simulink model "mavsim_chap10"  (R2020b)
settings: Solver=ode4  StartTime=0.0  StopTime=tsim  FixedStep=P.Ts  RelTol=1e-3  EnableMultiTasking=on
InitFcn:
  | param_chap10
values from neighbouring files (symbols this model uses):
  path_vector = [flag; r; q; chi_inf; k_path; c; rho; lambda; k_orbit]    [pathstruct2pathvec.m]    (also in runSim.m = pathstruct2pathvec(path_struct))
undefined symbols (not defined in the file or in its folder): accelerometer, aileron_c_sat, airspeed, baroAltimeter, calc_chi, closedLoopEnable, elevator_c_sat, forces_moments, get_h, get_p, get_phi, get_q, get_theta, get_Va, gps, gyro, magnetometer, P, phi_c_sat, stateMachine, takeoff_autopilot, theta_c_sat, throttle_c_sat, u_trim, x_trim
libraries: pid_lib x5, simulink x3
settings Model: Creator=beard  LastModifiedBy=alanf
settings DataIOCC: LimitDataPoints=on  SaveFormat=Array  ReturnWorkspaceOutputs=off
settings OptimizationCC: ExpressionDepthLimit=2147483647  InitFltsAndDblsToZero=on  LifeSpan=inf
settings DebuggingCC: UnderspecifiedInitializationDetection=Classic  MergeDetectMultiDrivingBlocksExec=none  SolverPrmCheckMsg=warning  FcnCallInpInsideContextMsg=warning  StateNameClashWarn=warning  SFUnexpectedBacktrackingDiag=warning  SFNoUnconditionalDefaultTransitionDiag=warning  SFExecutionAtInitializationDiag=none  ArithmeticOperatorsInVariantConditions=warning
settings HardwareCC: ProdBitPerPointer=32  ProdBitPerSizeT=32  ProdBitPerPtrDiffT=32  ProdLargestAtomicFloat=None  ProdIntDivRoundTo=Undefined  ProdEndianess=Unspecified  ProdWordSize=32  ProdHWDeviceType=32-bit Generic
settings ModelReferenceCC: PropagateSignalLabelsOutOfModel=off
settings SFSimCC: SimUseLocalCustomCode=off  CustomCodeUndefinedFunction=UseInterfaceOnly
settings RTWCC: RTWUseLocalCustomCode=off
settings CodeAppCC: StateflowObjectComments=on
settings GRTTargetCC: TargetLangStandard=C89/C90 (ANSI)  CombineOutputUpdateFcns=off  GRTInterface=on
settings ConfigComp: CovMetricSettings=dw  CovSaveCumulativeToWorkspaceVar=on  CovSaveSingleToWorkspaceVar=on  CovExternalEMLEnable=off  CovSFcnEnable=off

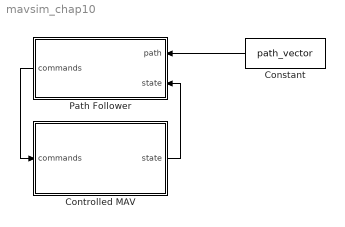
== system mavsim_chap10 ==
  Constant : Constant  Value=path_vector
  Controlled MAV : Subsystem
      mask Display: image(imread('batcam.png'))
  Path Follower : Subsystem
  wires:
  Controlled MAV/1(state) -> Path Follower/2(state)
  Path Follower/1(commands) -> Controlled MAV/1(commands)
  Constant/1 -> Path Follower/1(path)

== system mavsim_chap10/Controlled MAV ==
  commands : Inport
  Autopilot : Subsystem
      mask Display: image(imread('kestrel.jpg'))
  MAV : Subsystem
      mask Display: image(imread('batcam.png'))
  Wind : Subsystem
  state : Outport  VectorParamsAs1DForOutWhenUnconnected=off
  wires:
  Wind/1(Wind) -> MAV/2(wind)
  MAV/1(x) -> state/1, Autopilot/2(x)  "state"
  Autopilot/1(delta) -> MAV/1(delta)
  commands/1 -> Autopilot/1(commands)

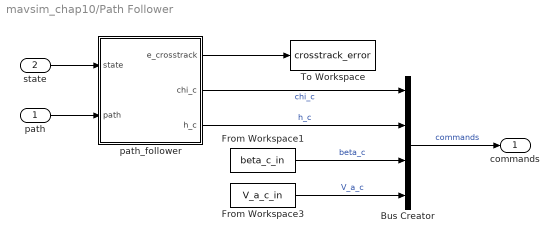
== system mavsim_chap10/Path Follower ==
  path : Inport
  state : Inport  Port=2
  Bus Creator : BusCreator  Inputs=4
  From Workspace1 : FromWorkspace  VariableName=beta_c_in
  From Workspace3 : FromWorkspace  VariableName=V_a_c_in
  To Workspace : ToWorkspace  VariableName=crosstrack_error  SaveFormat=Timeseries  SampleTime=-1
  path_follower : MATLAB Function  TreatAsAtomicUnit=on
  commands : Outport  VectorParamsAs1DForOutWhenUnconnected=off
  wires:
  From Workspace3/1 -> Bus Creator/4  "V_a_c"
  Bus Creator/1 -> commands/1  "commands"
  From Workspace1/1 -> Bus Creator/3  "beta_c"
  path_follower/2(chi_c) -> Bus Creator/1  "chi_c"
  path_follower/3(h_c) -> Bus Creator/2  "h_c"
  state/1 -> path_follower/1(state)
  path/1 -> path_follower/2(path)
  path_follower/1(e_crosstrack) -> To Workspace/1

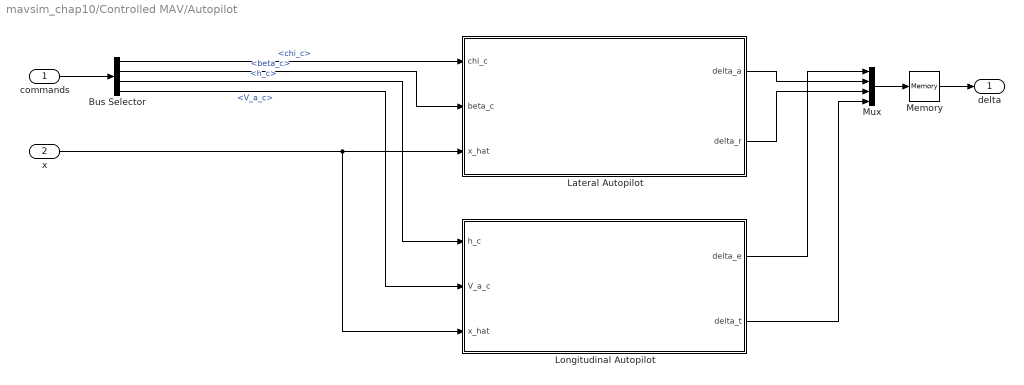
== system mavsim_chap10/Controlled MAV/Autopilot ==
  commands : Inport
  x : Inport  Port=2
  Bus Selector : BusSelector  OutputSignals=chi_c,beta_c,h_c,V_a_c
  Lateral Autopilot : Subsystem
  Longitudinal Autopilot : Subsystem
  Memory : Memory  InitialCondition=P.u_trim  InheritSampleTime=on
  Mux : Mux
  delta : Outport  VectorParamsAs1DForOutWhenUnconnected=off
  wires:
  x/1 -> Longitudinal Autopilot/3(x_hat), Lateral Autopilot/3(x_hat)
  Bus Selector/1 -> Lateral Autopilot/1(chi_c)  "<chi_c>"
  Bus Selector/2 -> Lateral Autopilot/2(beta_c)  "<beta_c>"
  Bus Selector/3 -> Longitudinal Autopilot/1(h_c)  "<h_c>"
  Bus Selector/4 -> Longitudinal Autopilot/2(V_a_c)  "<V_a_c>"
  Mux/1 -> Memory/1
  Memory/1 -> delta/1
  Longitudinal Autopilot/1(delta_e) -> Mux/1
  Lateral Autopilot/1(delta_a) -> Mux/2
  Lateral Autopilot/2(delta_r) -> Mux/3
  Longitudinal Autopilot/2(delta_t) -> Mux/4
  commands/1 -> Bus Selector/1

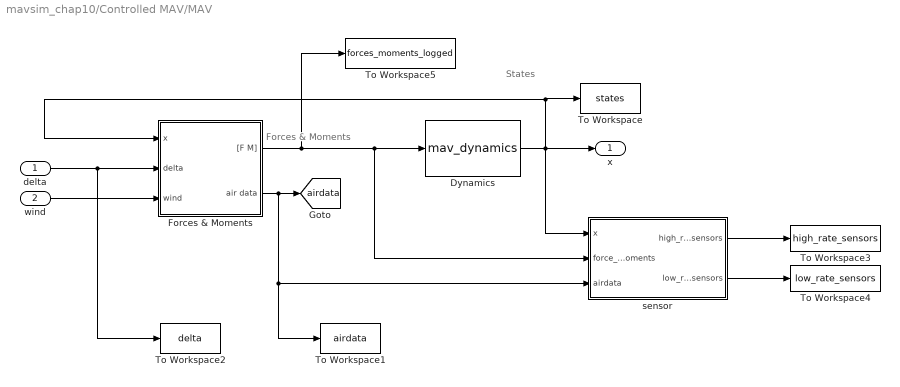
== system mavsim_chap10/Controlled MAV/MAV ==
  note: Forces & Moments
  note: States
  delta : Inport
  wind : Inport  Port=2
  Dynamics : S-Function  FunctionName=mav_dynamics  Parameters=P  SFunctionDeploymentMode=off  EnableBusSupport=off
  Forces & Moments : Subsystem
  To Workspace : ToWorkspace  VariableName=states  SaveFormat=Timeseries  SampleTime=-1
  To Workspace1 : ToWorkspace  VariableName=airdata  SaveFormat=Timeseries  SampleTime=-1
  To Workspace2 : ToWorkspace  VariableName=delta  SaveFormat=Timeseries  SampleTime=-1
  To Workspace3 : ToWorkspace  VariableName=high_rate_sensors  SaveFormat=Timeseries  SampleTime=-1
  To Workspace4 : ToWorkspace  VariableName=low_rate_sensors  SaveFormat=Timeseries  SampleTime=-1
  To Workspace5 : ToWorkspace  VariableName=forces_moments_logged  SaveFormat=Timeseries  SampleTime=-1
  sensor : Subsystem
  x : Outport  VectorParamsAs1DForOutWhenUnconnected=off
  tag scope: airdata=global
  wires:
  Dynamics/1 -> sensor/1(x), Forces & Moments/1(x), To Workspace/1, x/1
  Forces & Moments/1("[F M]") -> To Workspace5/1, sensor/2(force_moments), Dynamics/1
  Forces & Moments/2(air data) -> To Workspace1/1, sensor/3(airdata), [airdata]
  delta/1 -> To Workspace2/1, Forces & Moments/2(delta)
  wind/1 -> Forces & Moments/3(wind)
  sensor/1(high_rate_sensors) -> To Workspace3/1
  sensor/2(low_rate_sensors) -> To Workspace4/1

== system mavsim_chap10/Controlled MAV/Wind ==
  Constant2 : Constant  Value=[P.wind_n; P.wind_e; P.wind_d]
  Mux1 : Mux  Inputs=2
  Wind Gusts : Subsystem
  Wind : Outport  VectorParamsAs1DForOutWhenUnconnected=off
  wires:
  Constant2/1 -> Mux1/1
  Mux1/1 -> Wind/1
  Wind Gusts/1(gusts) -> Mux1/2

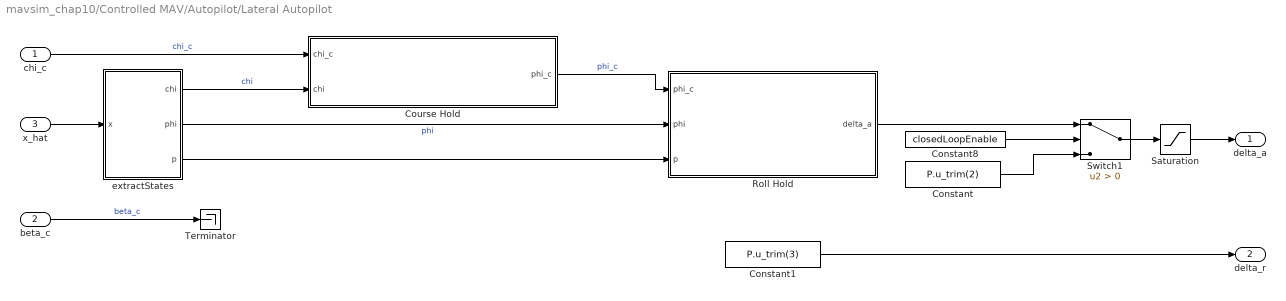
== system mavsim_chap10/Controlled MAV/Autopilot/Lateral Autopilot ==
  chi_c : Inport
  beta_c : Inport  Port=2
  x_hat : Inport  Port=3
  Constant : Constant  Value=P.u_trim(2)
  Constant1 : Constant  Value=P.u_trim(3)
  Constant8 : Constant  Value=closedLoopEnable
  Course Hold : Subsystem
  Roll Hold : Subsystem
  Saturation : Saturate  UpperLimit=aileron_c_sat  LowerLimit=-aileron_c_sat
  Switch1 : Switch  Criteria=u2 > Threshold
  Terminator : Terminator
  extractStates : Subsystem
  delta_a : Outport  VectorParamsAs1DForOutWhenUnconnected=off
  delta_r : Outport  Port=2  VectorParamsAs1DForOutWhenUnconnected=off
  wires:
  chi_c/1 -> Course Hold/1(chi_c)  "chi_c"
  Course Hold/1(phi_c) -> Roll Hold/1(phi_c)  "phi_c"
  x_hat/1 -> extractStates/1(x)
  extractStates/1(chi) -> Course Hold/2(chi)  "chi"
  extractStates/2(phi) -> Roll Hold/2(phi)  "phi"
  extractStates/3(p) -> Roll Hold/3(p)
  Constant1/1 -> delta_r/1
  Switch1/1 -> Saturation/1
  Constant/1 -> Switch1/3
  Roll Hold/1(delta_a) -> Switch1/1
  Constant8/1 -> Switch1/2
  beta_c/1 -> Terminator/1  "beta_c"
  Saturation/1 -> delta_a/1

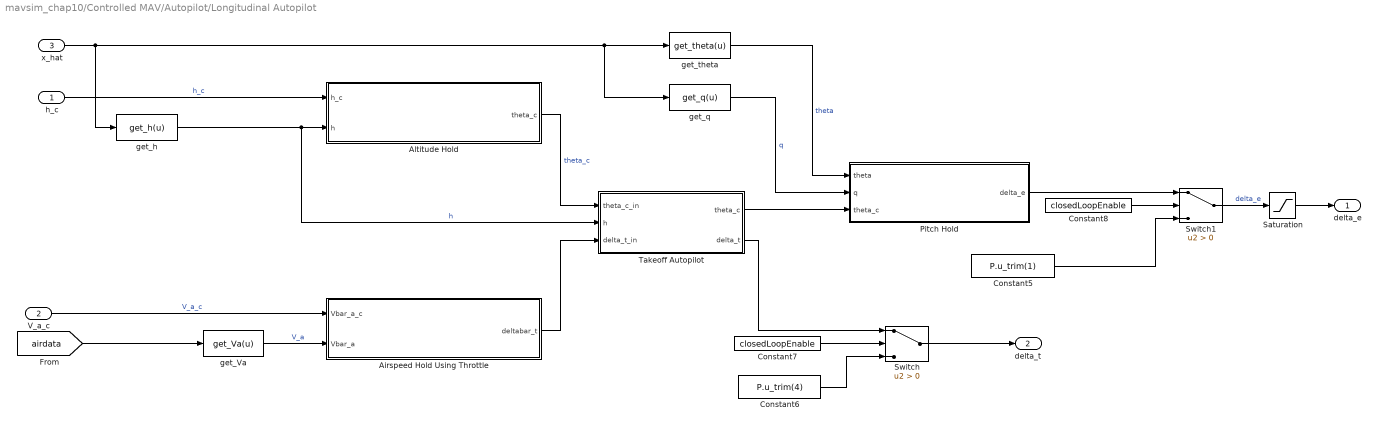
== system mavsim_chap10/Controlled MAV/Autopilot/Longitudinal Autopilot ==
  h_c : Inport
  V_a_c : Inport  Port=2
  x_hat : Inport  Port=3
  Airspeed Hold Using Throttle : Subsystem
  Altitude Hold : Subsystem
  Constant5 : Constant  Value=P.u_trim(1)
  Constant6 : Constant  Value=P.u_trim(4)
  Constant7 : Constant  Value=closedLoopEnable
  Constant8 : Constant  Value=closedLoopEnable
  Pitch Hold : Subsystem
  Saturation : Saturate  UpperLimit=elevator_c_sat  LowerLimit=-elevator_c_sat
  Switch : Switch  Criteria=u2 > Threshold
  Switch1 : Switch  Criteria=u2 > Threshold
  Takeoff Autopilot : Subsystem
  get_Va : MATLABFcn  MATLABFcn=get_Va(u)
  get_h : MATLABFcn  MATLABFcn=get_h(u)
  get_q : MATLABFcn  MATLABFcn=get_q(u)
  get_theta : MATLABFcn  MATLABFcn=get_theta(u)
  delta_e : Outport  VectorParamsAs1DForOutWhenUnconnected=off
  delta_t : Outport  Port=2  VectorParamsAs1DForOutWhenUnconnected=off
  wires:
  h_c/1 -> Altitude Hold/1(h_c)  "h_c"
  x_hat/1 -> get_q/1, get_theta/1, get_h/1
  get_h/1 -> Takeoff Autopilot/2(h), Altitude Hold/2(h)  "h"
  [airdata] -> get_Va/1
  get_Va/1 -> Airspeed Hold Using Throttle/2(Vbar_a)  "V_a"
  get_theta/1 -> Pitch Hold/1(theta)  "theta"
  get_q/1 -> Pitch Hold/2(q)  "q"
  Constant6/1 -> Switch/3
  Switch/1 -> delta_t/1
  Switch1/1 -> Saturation/1  "delta_e"
  Constant5/1 -> Switch1/3
  Constant7/1 -> Switch/2
  Constant8/1 -> Switch1/2
  V_a_c/1 -> Airspeed Hold Using Throttle/1(Vbar_a_c)  "V_a_c"
  Pitch Hold/1(delta_e) -> Switch1/1
  Saturation/1 -> delta_e/1
  Altitude Hold/1(theta_c) -> Takeoff Autopilot/1(theta_c_in)  "theta_c"
  Airspeed Hold Using Throttle/1(deltabar_t) -> Takeoff Autopilot/3(delta_t_in)
  Takeoff Autopilot/1(theta_c) -> Pitch Hold/3(theta_c)
  Takeoff Autopilot/2(delta_t) -> Switch/1

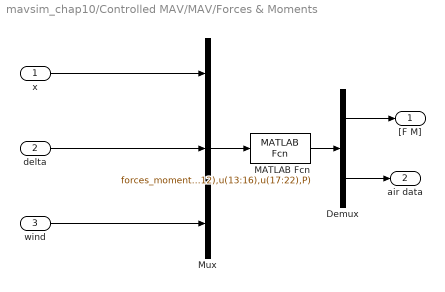
== system mavsim_chap10/Controlled MAV/MAV/Forces & Moments ==
  x : Inport
  delta : Inport  Port=2
  wind : Inport  Port=3
  Demux : Demux  Outputs=[6;6]
  MATLAB Fcn : MATLABFcn  MATLABFcn=forces_moments(u(1:12),u(13:16),u(17:22),P)  OutputDimensions=12
  Mux : Mux  Inputs=3
  "[F M]" : Outport  VectorParamsAs1DForOutWhenUnconnected=off
  air data : Outport  Port=2  VectorParamsAs1DForOutWhenUnconnected=off
  wires:
  Demux/2 -> air data/1
  Mux/1 -> MATLAB Fcn/1
  Demux/1 -> "[F M]"/1
  MATLAB Fcn/1 -> Demux/1
  wind/1 -> Mux/3
  delta/1 -> Mux/2
  x/1 -> Mux/1

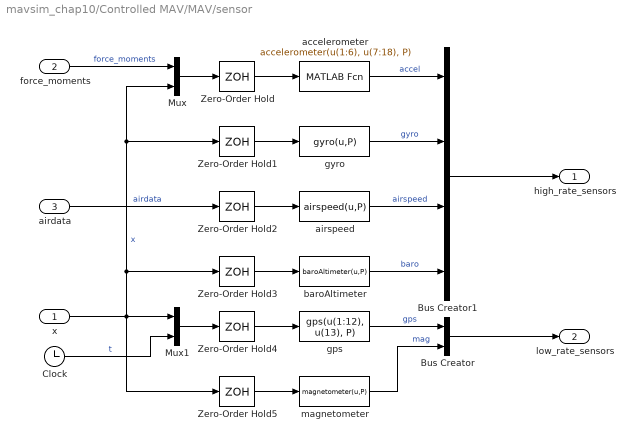
== system mavsim_chap10/Controlled MAV/MAV/sensor ==
  x : Inport
  force_moments : Inport  Port=2
  airdata : Inport  Port=3
  Bus Creator : BusCreator  Inputs=2
  Bus Creator1 : BusCreator  Inputs=4
  Clock : Clock
  Mux : Mux  Inputs=2
  Mux1 : Mux  Inputs=2
  Zero-Order Hold{,1..3} (4 alike) : ZeroOrderHold  SampleTime=P.Ts_highrate
  Zero-Order Hold4 : ZeroOrderHold  SampleTime=P.Ts_lowrate
  Zero-Order Hold5 : ZeroOrderHold  SampleTime=P.Ts_lowrate
  accelerometer : MATLABFcn  MATLABFcn=accelerometer(u(1:6), u(7:18), P)
  airspeed : MATLABFcn  MATLABFcn=airspeed(u,P)
  baroAltimeter : MATLABFcn  MATLABFcn=baroAltimeter(u,P)
  gps : MATLABFcn  MATLABFcn=gps(u(1:12), u(13), P)
  gyro : MATLABFcn  MATLABFcn=gyro(u,P)
  magnetometer : MATLABFcn  MATLABFcn=magnetometer(u,P)
  high_rate_sensors : Outport  VectorParamsAs1DForOutWhenUnconnected=off
  low_rate_sensors : Outport  Port=2  VectorParamsAs1DForOutWhenUnconnected=off
  wires:
  gps/1 -> Bus Creator/1  "gps"
  magnetometer/1 -> Bus Creator/2  "mag"
  Bus Creator/1 -> low_rate_sensors/1
  x/1 -> Mux1/1, Mux/2, Zero-Order Hold1/1, Zero-Order Hold3/1, Zero-Order Hold5/1  "x"
  airdata/1 -> Zero-Order Hold2/1  "airdata"
  accelerometer/1 -> Bus Creator1/1  "accel"
  gyro/1 -> Bus Creator1/2  "gyro"
  airspeed/1 -> Bus Creator1/3  "airspeed"
  baroAltimeter/1 -> Bus Creator1/4  "baro"
  Bus Creator1/1 -> high_rate_sensors/1
  Clock/1 -> Mux1/2  "t"
  Zero-Order Hold/1 -> accelerometer/1
  Zero-Order Hold1/1 -> gyro/1
  Zero-Order Hold2/1 -> airspeed/1
  Zero-Order Hold3/1 -> baroAltimeter/1
  Zero-Order Hold4/1 -> gps/1
  Zero-Order Hold5/1 -> magnetometer/1
  force_moments/1 -> Mux/1  "force_moments"
  Mux/1 -> Zero-Order Hold/1
  Mux1/1 -> Zero-Order Hold4/1

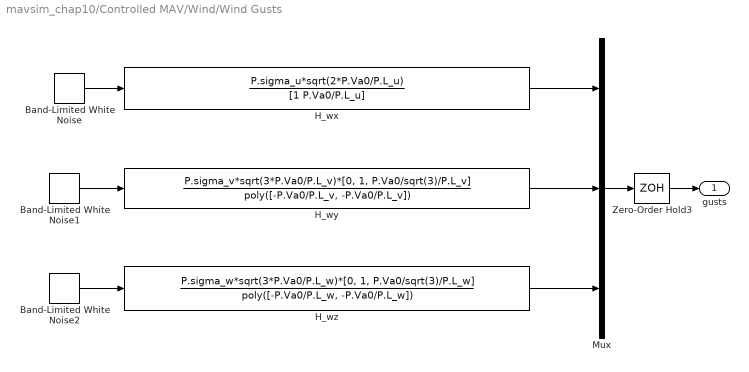
== system mavsim_chap10/Controlled MAV/Wind/Wind Gusts ==
  Band-Limited White Noise : simulink/Sources/Band-Limited White Noise  Cov=[1]  Ts=P.Ts  seed=[23341]
  Band-Limited White Noise1 : simulink/Sources/Band-Limited White Noise  Cov=[1]  Ts=P.Ts  seed=[23341]
  Band-Limited White Noise2 : simulink/Sources/Band-Limited White Noise  Cov=[1]  Ts=P.Ts  seed=[23341]
  H_wx : TransferFcn  Numerator=P.sigma_u*sqrt(2*P.Va0/P.L_u)  Denominator=[1 P.Va0/P.L_u]
  H_wy : TransferFcn  Numerator=P.sigma_v*sqrt(3*P.Va0/P.L_v)*[0, 1, P.Va0/sqrt(3)/P.L_v]  Denominator=poly([-P.Va0/P.L_v, -P.Va0/P.L_v])
  H_wz : TransferFcn  Numerator=P.sigma_w*sqrt(3*P.Va0/P.L_w)*[0, 1, P.Va0/sqrt(3)/P.L_w]  Denominator=poly([-P.Va0/P.L_w, -P.Va0/P.L_w])
  Mux : Mux  Inputs=3
  Zero-Order Hold3 : ZeroOrderHold  SampleTime=P.Ts
  gusts : Outport  VectorParamsAs1DForOutWhenUnconnected=off
  wires:
  H_wx/1 -> Mux/1
  Band-Limited White Noise/1 -> H_wx/1
  H_wy/1 -> Mux/2
  Band-Limited White Noise1/1 -> H_wy/1
  H_wz/1 -> Mux/3
  Band-Limited White Noise2/1 -> H_wz/1
  Mux/1 -> Zero-Order Hold3/1
  Zero-Order Hold3/1 -> gusts/1

== system mavsim_chap10/Controlled MAV/Autopilot/Lateral Autopilot/Course Hold ==
  chi_c : Inport
  chi : Inport  Port=2
  PI Controller : pid_lib/PID Controller  Controller=PI  Form=Parallel  TimeDomain=Continuous-time  UseExternalTs=off  SampleTime=-1  IntegratorMethod=Forward Euler  FilterMethod=Forward Euler  ControllerParametersSource=internal  P=P.k_pchi  I=P.k_ichi  D=0  UseFilter=on  N=100  TunerSelectOption=Transfer Function Based (PID Tuner App)  InitialConditionSource=internal  InitialConditionForIntegrator=x_trim(7)  InitialConditionForFilter=0  DifferentiatorICPrevScaledInput=0  ExternalReset=none  TrackingMode=off  Kt=1  LimitOutput=on  SatLimitsSource=internal  UpperSaturationLimit=phi_c_sat  LowerSaturationLimit=-phi_c_sat  LinearizeAsGain=off  AntiWindupMode=clamping  Kb=1  POutMin=[]  POutMax=[]  IOutMin=[]  IOutMax=[]  DOutMin=[]  DOutMax=[]  NOutMin=[]  NOutMax=[]  SumOutMin=[]  SumOutMax=[]  SaturationOutMin=[]  SaturationOutMax=[]  PParamMin=[]  PParamMax=[]  IParamMin=[]  IParamMax=[]  DParamMin=[]  DParamMax=[]  NParamMin=[]  NParamMax=[]  KbParamMin=[]  KbParamMax=[]  KtParamMin=[]  KtParamMax=[]  KbOutMin=[]  KbOutMax=[]  KtOutMin=[]  KtOutMax=[]  IntegratorOutMin=[]  IntegratorOutMax=[]  FilterOutMin=[]  FilterOutMax=[]  SumI1OutMin=[]  SumI1OutMax=[]  SumI2OutMin=[]  SumI2OutMax=[]  SumI3OutMin=[]  SumI3OutMax=[]  SumI4OutMin=[]  SumI4OutMax=[]  SumDOutMin=[]  SumDOutMax=[]  DifferentiatorOutMin=[]  DifferentiatorOutMax=[]  FilterDiffOutCoefMin=[]  FilterDiffOutCoefMax=[]  ReciprocalOutMin=[]  ReciprocalOutMax=[]  SumDenOutMin=[]  SumDenOutMax=[]  SumNumOutMin=[]  SumNumOutMax=[]  DivideOutMin=[]  DivideOutMax=[]  UdiffTsProdOutMin=[]  UdiffTsProdOutMax=[]  NTsProdOutMin=[]  NTsProdOutMax=[]  UintegralTsProdOutMin=[]  UintegralTsProdOutMax=[]  UngainTsProdOutMin=[]  UngainTsProdOutMax=[]  IntegratorContinuousStateAttributes=''  IntegratorStateMustResolveToSignalObject=off  IntegratorRTWStateStorageClass=Auto  FilterContinuousStateAttributes=''  FilterStateMustResolveToSignalObject=off  FilterRTWStateStorageClass=Auto  ParallelPVariant=InternalParameters  IdealPVariant=Disabled  IVariant=InternalParameters  DVariant=Disabled  IntegratorVariant=Continuous  SatVariant=Enabled  AWVariant=ContClampingParallel  PCopyVariant=Disabled  TRVariant=Disabled  FdbkBlocksVariant=Forward  IdealPFdbkVariant=Disabled  SatFdbkVariant=Disabled  DerivativeFilterVariant=Disabled  NVariant=Disabled  NCopyVariant=Disabled_SignalSpec  FilterICVariant=Disabled  IntegratorICVariant=InternalICs  ExternalResetVariant=Disabled  TRSumVariant=Passthrough  SumFdbkVariant=Disabled  SumVariant=Sum_PI  TsampFilterVariant=InternalTs  TsampNgainVariant=Passthrough  TsampIntegralVariant=Passthrough  ExternalSaturationOutDataTypeStr=Inherit: Same as second input
  Sum1 : Sum  Inputs=|+-
  To Workspace : ToWorkspace  VariableName=chi_c  SaveFormat=Timeseries  SampleTime=-1
  To Workspace1 : ToWorkspace  VariableName=chi  SaveFormat=Timeseries  SampleTime=-1
  phi_c : Outport  VectorParamsAs1DForOutWhenUnconnected=off
  wires:
  chi/1 -> To Workspace1/1, Sum1/2  "chi"
  chi_c/1 -> To Workspace/1, Sum1/1  "chi_c"
  Sum1/1 -> PI Controller/1  "e_chi"
  PI Controller/1 -> phi_c/1

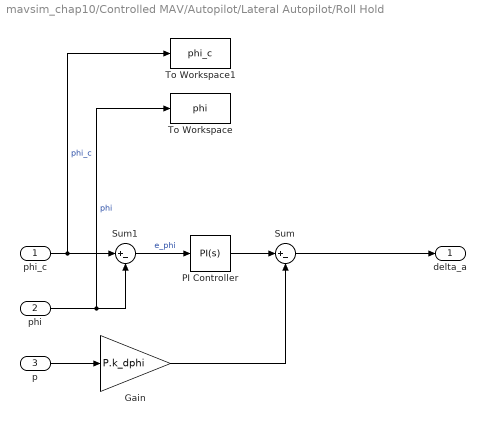
== system mavsim_chap10/Controlled MAV/Autopilot/Lateral Autopilot/Roll Hold ==
  phi_c : Inport
  phi : Inport  Port=2
  p : Inport  Port=3
  Gain : Gain  Gain=P.k_dphi
  PI Controller : pid_lib/PID Controller  Controller=PI  Form=Parallel  TimeDomain=Continuous-time  UseExternalTs=off  SampleTime=-1  IntegratorMethod=Forward Euler  FilterMethod=Forward Euler  ControllerParametersSource=internal  P=P.k_pphi  I=P.k_iphi  D=0  UseFilter=on  N=100  TunerSelectOption=Transfer Function Based (PID Tuner App)  InitialConditionSource=internal  InitialConditionForIntegrator=u_trim(2)  InitialConditionForFilter=0  DifferentiatorICPrevScaledInput=0  ExternalReset=none  TrackingMode=off  Kt=1  LimitOutput=off  SatLimitsSource=internal  UpperSaturationLimit=inf  LowerSaturationLimit=-inf  LinearizeAsGain=on  AntiWindupMode=clamping  Kb=1  POutMin=[]  POutMax=[]  IOutMin=[]  IOutMax=[]  DOutMin=[]  DOutMax=[]  NOutMin=[]  NOutMax=[]  SumOutMin=[]  SumOutMax=[]  SaturationOutMin=[]  SaturationOutMax=[]  PParamMin=[]  PParamMax=[]  IParamMin=[]  IParamMax=[]  DParamMin=[]  DParamMax=[]  NParamMin=[]  NParamMax=[]  KbParamMin=[]  KbParamMax=[]  KtParamMin=[]  KtParamMax=[]  KbOutMin=[]  KbOutMax=[]  KtOutMin=[]  KtOutMax=[]  IntegratorOutMin=[]  IntegratorOutMax=[]  FilterOutMin=[]  FilterOutMax=[]  SumI1OutMin=[]  SumI1OutMax=[]  SumI2OutMin=[]  SumI2OutMax=[]  SumI3OutMin=[]  SumI3OutMax=[]  SumI4OutMin=[]  SumI4OutMax=[]  SumDOutMin=[]  SumDOutMax=[]  DifferentiatorOutMin=[]  DifferentiatorOutMax=[]  FilterDiffOutCoefMin=[]  FilterDiffOutCoefMax=[]  ReciprocalOutMin=[]  ReciprocalOutMax=[]  SumDenOutMin=[]  SumDenOutMax=[]  SumNumOutMin=[]  SumNumOutMax=[]  DivideOutMin=[]  DivideOutMax=[]  UdiffTsProdOutMin=[]  UdiffTsProdOutMax=[]  NTsProdOutMin=[]  NTsProdOutMax=[]  UintegralTsProdOutMin=[]  UintegralTsProdOutMax=[]  UngainTsProdOutMin=[]  UngainTsProdOutMax=[]  IntegratorContinuousStateAttributes=''  IntegratorStateMustResolveToSignalObject=off  IntegratorRTWStateStorageClass=Auto  FilterContinuousStateAttributes=''  FilterStateMustResolveToSignalObject=off  FilterRTWStateStorageClass=Auto  ParallelPVariant=InternalParameters  IdealPVariant=Disabled  IVariant=InternalParameters  DVariant=Disabled  IntegratorVariant=Continuous  SatVariant=Disabled  AWVariant=Passthrough  PCopyVariant=Disabled  TRVariant=Disabled  FdbkBlocksVariant=Forward  IdealPFdbkVariant=Disabled  SatFdbkVariant=Disabled  DerivativeFilterVariant=Disabled  NVariant=Disabled  NCopyVariant=Disabled_SignalSpec  FilterICVariant=Disabled  IntegratorICVariant=InternalICs  ExternalResetVariant=Disabled  TRSumVariant=Passthrough  SumFdbkVariant=Disabled  SumVariant=Sum_PI  TsampFilterVariant=InternalTs  TsampNgainVariant=Passthrough  TsampIntegralVariant=Passthrough  ExternalSaturationOutDataTypeStr=Inherit: Same as second input
  Sum : Sum  Inputs=|+-
  Sum1 : Sum  Inputs=|+-
  To Workspace : ToWorkspace  VariableName=phi  SaveFormat=Timeseries  SampleTime=-1
  To Workspace1 : ToWorkspace  VariableName=phi_c  SaveFormat=Timeseries  SampleTime=-1
  delta_a : Outport  VectorParamsAs1DForOutWhenUnconnected=off
  wires:
  Sum1/1 -> PI Controller/1  "e_phi"
  phi_c/1 -> To Workspace1/1, Sum1/1  "phi_c"
  PI Controller/1 -> Sum/1
  phi/1 -> To Workspace/1, Sum1/2  "phi"
  p/1 -> Gain/1
  Gain/1 -> Sum/2
  Sum/1 -> delta_a/1

== system mavsim_chap10/Controlled MAV/Autopilot/Lateral Autopilot/extractStates ==
  x : Inport
  calc_chi : MATLABFcn  MATLABFcn=calc_chi(u)
  get_p : MATLABFcn  MATLABFcn=get_p(u)
  get_phi : MATLABFcn  MATLABFcn=get_phi(u)
  chi : Outport  VectorParamsAs1DForOutWhenUnconnected=off
  phi : Outport  Port=2  VectorParamsAs1DForOutWhenUnconnected=off
  p : Outport  Port=3  VectorParamsAs1DForOutWhenUnconnected=off
  wires:
  x/1 -> get_p/1, get_phi/1, calc_chi/1
  calc_chi/1 -> chi/1
  get_phi/1 -> phi/1
  get_p/1 -> p/1

== system mavsim_chap10/Controlled MAV/Autopilot/Longitudinal Autopilot/Airspeed Hold Using Throttle ==
  Vbar_a_c : Inport
  Vbar_a : Inport  Port=2
  PI Controller : pid_lib/PID Controller  Controller=PI  Form=Parallel  TimeDomain=Continuous-time  UseExternalTs=off  SampleTime=-1  IntegratorMethod=Forward Euler  FilterMethod=Forward Euler  ControllerParametersSource=internal  P=P.k_pv  I=P.k_iv  D=0  UseFilter=on  N=100  TunerSelectOption=Transfer Function Based (PID Tuner App)  InitialConditionSource=internal  InitialConditionForIntegrator=P.u_trim(4)  InitialConditionForFilter=0  DifferentiatorICPrevScaledInput=0  ExternalReset=none  TrackingMode=off  Kt=1  LimitOutput=on  SatLimitsSource=internal  UpperSaturationLimit=throttle_c_sat  LowerSaturationLimit=0  LinearizeAsGain=on  AntiWindupMode=clamping  Kb=1  POutMin=[]  POutMax=[]  IOutMin=[]  IOutMax=[]  DOutMin=[]  DOutMax=[]  NOutMin=[]  NOutMax=[]  SumOutMin=[]  SumOutMax=[]  SaturationOutMin=[]  SaturationOutMax=[]  PParamMin=[]  PParamMax=[]  IParamMin=[]  IParamMax=[]  DParamMin=[]  DParamMax=[]  NParamMin=[]  NParamMax=[]  KbParamMin=[]  KbParamMax=[]  KtParamMin=[]  KtParamMax=[]  KbOutMin=[]  KbOutMax=[]  KtOutMin=[]  KtOutMax=[]  IntegratorOutMin=[]  IntegratorOutMax=[]  FilterOutMin=[]  FilterOutMax=[]  SumI1OutMin=[]  SumI1OutMax=[]  SumI2OutMin=[]  SumI2OutMax=[]  SumI3OutMin=[]  SumI3OutMax=[]  SumI4OutMin=[]  SumI4OutMax=[]  SumDOutMin=[]  SumDOutMax=[]  DifferentiatorOutMin=[]  DifferentiatorOutMax=[]  FilterDiffOutCoefMin=[]  FilterDiffOutCoefMax=[]  ReciprocalOutMin=[]  ReciprocalOutMax=[]  SumDenOutMin=[]  SumDenOutMax=[]  SumNumOutMin=[]  SumNumOutMax=[]  DivideOutMin=[]  DivideOutMax=[]  UdiffTsProdOutMin=[]  UdiffTsProdOutMax=[]  NTsProdOutMin=[]  NTsProdOutMax=[]  UintegralTsProdOutMin=[]  UintegralTsProdOutMax=[]  UngainTsProdOutMin=[]  UngainTsProdOutMax=[]  IntegratorContinuousStateAttributes=''  IntegratorStateMustResolveToSignalObject=off  IntegratorRTWStateStorageClass=Auto  FilterContinuousStateAttributes=''  FilterStateMustResolveToSignalObject=off  FilterRTWStateStorageClass=Auto  ParallelPVariant=InternalParameters  IdealPVariant=Disabled  IVariant=InternalParameters  DVariant=Disabled  IntegratorVariant=Continuous  SatVariant=Enabled  AWVariant=ContClampingParallel  PCopyVariant=Disabled  TRVariant=Disabled  FdbkBlocksVariant=Forward  IdealPFdbkVariant=Disabled  SatFdbkVariant=Disabled  DerivativeFilterVariant=Disabled  NVariant=Disabled  NCopyVariant=Disabled_SignalSpec  FilterICVariant=Disabled  IntegratorICVariant=InternalICs  ExternalResetVariant=Disabled  TRSumVariant=Passthrough  SumFdbkVariant=Disabled  SumVariant=Sum_PI  TsampFilterVariant=InternalTs  TsampNgainVariant=Passthrough  TsampIntegralVariant=Passthrough  ExternalSaturationOutDataTypeStr=Inherit: Same as second input
  Sum1 : Sum  Inputs=|+-
  To Workspace : ToWorkspace  VariableName=Vbar_a_c  SaveFormat=Timeseries  SampleTime=-1
  To Workspace1 : ToWorkspace  VariableName=Vbar_a  SaveFormat=Timeseries  SampleTime=-1
  deltabar_t : Outport  VectorParamsAs1DForOutWhenUnconnected=off
  wires:
  Sum1/1 -> PI Controller/1
  Vbar_a_c/1 -> To Workspace/1, Sum1/1
  Vbar_a/1 -> To Workspace1/1, Sum1/2
  PI Controller/1 -> deltabar_t/1

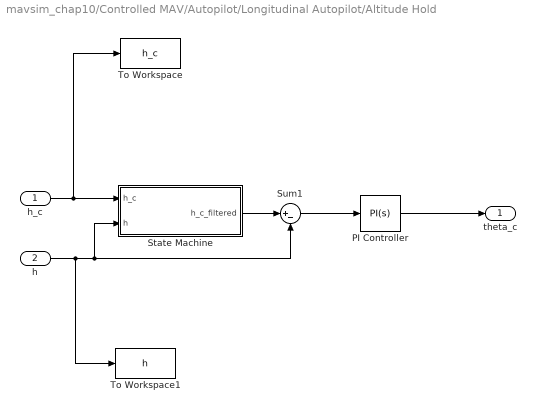
== system mavsim_chap10/Controlled MAV/Autopilot/Longitudinal Autopilot/Altitude Hold ==
  h_c : Inport
  h : Inport  Port=2
  PI Controller : pid_lib/PID Controller  Controller=PI  Form=Parallel  TimeDomain=Continuous-time  UseExternalTs=off  SampleTime=-1  IntegratorMethod=Forward Euler  FilterMethod=Forward Euler  ControllerParametersSource=internal  P=P.k_ph  I=P.k_ih  D=0  UseFilter=on  N=100  TunerSelectOption=Transfer Function Based (PID Tuner App)  InitialConditionSource=internal  InitialConditionForIntegrator=x_trim(8)  InitialConditionForFilter=0  DifferentiatorICPrevScaledInput=0  ExternalReset=none  TrackingMode=off  Kt=1  LimitOutput=on  SatLimitsSource=internal  UpperSaturationLimit=theta_c_sat  LowerSaturationLimit=-theta_c_sat  LinearizeAsGain=on  AntiWindupMode=clamping  Kb=1  POutMin=[]  POutMax=[]  IOutMin=[]  IOutMax=[]  DOutMin=[]  DOutMax=[]  NOutMin=[]  NOutMax=[]  SumOutMin=[]  SumOutMax=[]  SaturationOutMin=[]  SaturationOutMax=[]  PParamMin=[]  PParamMax=[]  IParamMin=[]  IParamMax=[]  DParamMin=[]  DParamMax=[]  NParamMin=[]  NParamMax=[]  KbParamMin=[]  KbParamMax=[]  KtParamMin=[]  KtParamMax=[]  KbOutMin=[]  KbOutMax=[]  KtOutMin=[]  KtOutMax=[]  IntegratorOutMin=[]  IntegratorOutMax=[]  FilterOutMin=[]  FilterOutMax=[]  SumI1OutMin=[]  SumI1OutMax=[]  SumI2OutMin=[]  SumI2OutMax=[]  SumI3OutMin=[]  SumI3OutMax=[]  SumI4OutMin=[]  SumI4OutMax=[]  SumDOutMin=[]  SumDOutMax=[]  DifferentiatorOutMin=[]  DifferentiatorOutMax=[]  FilterDiffOutCoefMin=[]  FilterDiffOutCoefMax=[]  ReciprocalOutMin=[]  ReciprocalOutMax=[]  SumDenOutMin=[]  SumDenOutMax=[]  SumNumOutMin=[]  SumNumOutMax=[]  DivideOutMin=[]  DivideOutMax=[]  UdiffTsProdOutMin=[]  UdiffTsProdOutMax=[]  NTsProdOutMin=[]  NTsProdOutMax=[]  UintegralTsProdOutMin=[]  UintegralTsProdOutMax=[]  UngainTsProdOutMin=[]  UngainTsProdOutMax=[]  IntegratorContinuousStateAttributes=''  IntegratorStateMustResolveToSignalObject=off  IntegratorRTWStateStorageClass=Auto  FilterContinuousStateAttributes=''  FilterStateMustResolveToSignalObject=off  FilterRTWStateStorageClass=Auto  ParallelPVariant=InternalParameters  IdealPVariant=Disabled  IVariant=InternalParameters  DVariant=Disabled  IntegratorVariant=Continuous  SatVariant=Enabled  AWVariant=ContClampingParallel  PCopyVariant=Disabled  TRVariant=Disabled  FdbkBlocksVariant=Forward  IdealPFdbkVariant=Disabled  SatFdbkVariant=Disabled  DerivativeFilterVariant=Disabled  NVariant=Disabled  NCopyVariant=Disabled_SignalSpec  FilterICVariant=Disabled  IntegratorICVariant=InternalICs  ExternalResetVariant=Disabled  TRSumVariant=Passthrough  SumFdbkVariant=Disabled  SumVariant=Sum_PI  TsampFilterVariant=InternalTs  TsampNgainVariant=Passthrough  TsampIntegralVariant=Passthrough  ExternalSaturationOutDataTypeStr=Inherit: Same as second input
  State Machine : Subsystem
  Sum1 : Sum  Inputs=|+-
  To Workspace : ToWorkspace  VariableName=h_c  SaveFormat=Timeseries  SampleTime=-1
  To Workspace1 : ToWorkspace  VariableName=h  SaveFormat=Timeseries  SampleTime=-1
  theta_c : Outport  VectorParamsAs1DForOutWhenUnconnected=off
  wires:
  Sum1/1 -> PI Controller/1
  h_c/1 -> To Workspace/1, State Machine/1(h_c)
  h/1 -> To Workspace1/1, State Machine/2(h), Sum1/2
  PI Controller/1 -> theta_c/1
  State Machine/1(h_c_filtered) -> Sum1/1

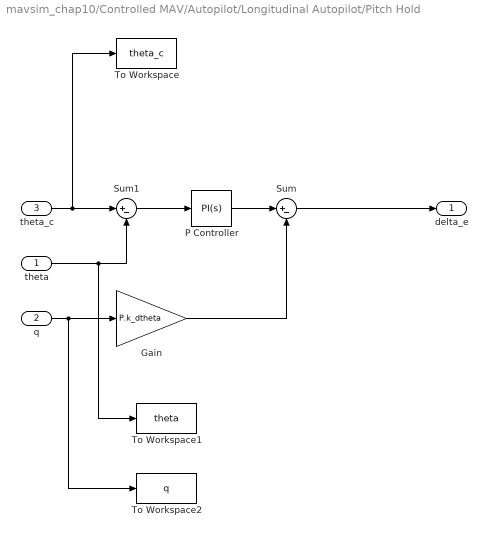
== system mavsim_chap10/Controlled MAV/Autopilot/Longitudinal Autopilot/Pitch Hold ==
  theta : Inport
  q : Inport  Port=2
  theta_c : Inport  Port=3
  Gain : Gain  Gain=P.k_dtheta
  P Controller : pid_lib/PID Controller  Controller=PI  Form=Parallel  TimeDomain=Continuous-time  UseExternalTs=off  SampleTime=-1  IntegratorMethod=Forward Euler  FilterMethod=Forward Euler  ControllerParametersSource=internal  P=P.k_ptheta  I=0  D=0  UseFilter=on  N=100  TunerSelectOption=Transfer Function Based (PID Tuner App)  InitialConditionSource=internal  InitialConditionForIntegrator=P.u_trim(1)  InitialConditionForFilter=0  DifferentiatorICPrevScaledInput=0  ExternalReset=none  TrackingMode=off  Kt=1  LimitOutput=off  SatLimitsSource=internal  UpperSaturationLimit=inf  LowerSaturationLimit=-inf  LinearizeAsGain=on  AntiWindupMode=clamping  Kb=1  POutMin=[]  POutMax=[]  IOutMin=[]  IOutMax=[]  DOutMin=[]  DOutMax=[]  NOutMin=[]  NOutMax=[]  SumOutMin=[]  SumOutMax=[]  SaturationOutMin=[]  SaturationOutMax=[]  PParamMin=[]  PParamMax=[]  IParamMin=[]  IParamMax=[]  DParamMin=[]  DParamMax=[]  NParamMin=[]  NParamMax=[]  KbParamMin=[]  KbParamMax=[]  KtParamMin=[]  KtParamMax=[]  KbOutMin=[]  KbOutMax=[]  KtOutMin=[]  KtOutMax=[]  IntegratorOutMin=[]  IntegratorOutMax=[]  FilterOutMin=[]  FilterOutMax=[]  SumI1OutMin=[]  SumI1OutMax=[]  SumI2OutMin=[]  SumI2OutMax=[]  SumI3OutMin=[]  SumI3OutMax=[]  SumI4OutMin=[]  SumI4OutMax=[]  SumDOutMin=[]  SumDOutMax=[]  DifferentiatorOutMin=[]  DifferentiatorOutMax=[]  FilterDiffOutCoefMin=[]  FilterDiffOutCoefMax=[]  ReciprocalOutMin=[]  ReciprocalOutMax=[]  SumDenOutMin=[]  SumDenOutMax=[]  SumNumOutMin=[]  SumNumOutMax=[]  DivideOutMin=[]  DivideOutMax=[]  UdiffTsProdOutMin=[]  UdiffTsProdOutMax=[]  NTsProdOutMin=[]  NTsProdOutMax=[]  UintegralTsProdOutMin=[]  UintegralTsProdOutMax=[]  UngainTsProdOutMin=[]  UngainTsProdOutMax=[]  IntegratorContinuousStateAttributes=''  IntegratorStateMustResolveToSignalObject=off  IntegratorRTWStateStorageClass=Auto  FilterContinuousStateAttributes=''  FilterStateMustResolveToSignalObject=off  FilterRTWStateStorageClass=Auto  ParallelPVariant=InternalParameters  IdealPVariant=Disabled  IVariant=InternalParameters  DVariant=Disabled  IntegratorVariant=Continuous  SatVariant=Disabled  AWVariant=Passthrough  PCopyVariant=Disabled  TRVariant=Disabled  FdbkBlocksVariant=Forward  IdealPFdbkVariant=Disabled  SatFdbkVariant=Disabled  DerivativeFilterVariant=Disabled  NVariant=Disabled  NCopyVariant=Disabled_SignalSpec  FilterICVariant=Disabled  IntegratorICVariant=InternalICs  ExternalResetVariant=Disabled  TRSumVariant=Passthrough  SumFdbkVariant=Disabled  SumVariant=Sum_PI  TsampFilterVariant=InternalTs  TsampNgainVariant=Passthrough  TsampIntegralVariant=Passthrough  ExternalSaturationOutDataTypeStr=Inherit: Same as second input
  Sum : Sum  Inputs=|+-
  Sum1 : Sum  Inputs=|+-
  To Workspace : ToWorkspace  VariableName=theta_c  SaveFormat=Timeseries  SampleTime=-1
  To Workspace1 : ToWorkspace  VariableName=theta  SaveFormat=Timeseries  SampleTime=-1
  To Workspace2 : ToWorkspace  VariableName=q  SaveFormat=Timeseries  SampleTime=-1
  delta_e : Outport  VectorParamsAs1DForOutWhenUnconnected=off
  wires:
  theta/1 -> To Workspace1/1, Sum1/2
  P Controller/1 -> Sum/1
  theta_c/1 -> To Workspace/1, Sum1/1
  Sum1/1 -> P Controller/1
  q/1 -> To Workspace2/1, Gain/1
  Gain/1 -> Sum/2
  Sum/1 -> delta_e/1

== system mavsim_chap10/Controlled MAV/Autopilot/Longitudinal Autopilot/Takeoff Autopilot ==
  theta_c_in : Inport
  h : Inport  Port=2
  delta_t_in : Inport  Port=3
  Demux : Demux  Outputs=2
  Mux : Mux  Inputs=3
  Takeoff Autopilot : MATLABFcn  MATLABFcn=takeoff_autopilot(u(1), u(2), u(3), P)  OutputDimensions=2  OutputSignalType=real
  theta_c : Outport  VectorParamsAs1DForOutWhenUnconnected=off
  delta_t : Outport  Port=2  VectorParamsAs1DForOutWhenUnconnected=off
  wires:
  h/1 -> Mux/2
  theta_c_in/1 -> Mux/1
  delta_t_in/1 -> Mux/3
  Mux/1 -> Takeoff Autopilot/1
  Takeoff Autopilot/1 -> Demux/1
  Demux/1 -> theta_c/1
  Demux/2 -> delta_t/1

== system mavsim_chap10/Controlled MAV/Autopilot/Longitudinal Autopilot/Altitude Hold/State Machine ==
  h_c : Inport
  h : Inport  Port=2
  Interpreted MATLAB Function : MATLABFcn  MATLABFcn=stateMachine(u(1), u(2), P)
  Mux : Mux  Inputs=2
  h_c_filtered : Outport  VectorParamsAs1DForOutWhenUnconnected=off
  wires:
  Interpreted MATLAB Function/1 -> h_c_filtered/1
  h_c/1 -> Mux/1
  h/1 -> Mux/2
  Mux/1 -> Interpreted MATLAB Function/1

== matlab function mavsim_chap10/Path Follower/path_follower ==
  data: e_crosstrack output; state input; path input; chi_c output size=1; h_c output size=1
function [e_crosstrack, chi_c, h_c] = fcn(state,path)
%% Create the path structure
path_struct = pathvec2pathstruct(path);

center = path_struct.center;
chi = calc_chi(state);
q = path_struct.direction;
r = path_struct.origin;
p = state(1:3);
k_path = path_struct.k_path;
chi_inf = path_struct.chi_inf;
k_orbit = path_struct.k_orbit;
radius = path_struct.radius;
orbit_direction = path_struct.orbit_direction;


% q = [qn; qe; qd]
% o = [on; oe; od]
% p = [pn; pe; pd]


if strcmp(path_struct.type,'lin')
    % Implement the straight line path follower
    % Algorithm 3
    chi_q = atan2(q(2), q(1));
% % %     dcm = [cos(chi_q) sin(chi_q) 0;
% % %            -sin(chi_q) cos(chi_q) 0;
% % %            0 0 1];
    e_p = (p-r);
% % %     e_p = dcm * e_p;
    
    k = [0; 0; 1];
    
    n = cross(q,k)/norm(cross(q,k));
    
    testn = n';
    test = e_p*testn;
    test = test*n;
    s = e_p - dot(e_p,n)*n;
    % s = [sn; se; sd]
    
    h_c = -r(3) - sqrt(s(1)^2 + s(2)^2)*(q(3)/sqrt(q(1)^2 + q(2)^2));

    while chi_q - chi < -pi
        chi_q = chi_q + 2*pi;
        break
    end
    while chi_q - chi > pi
        chi_q = chi_q - 2*pi;
        break
    end
    e_crosstrack = -sin(chi_q)*(p(1) - r(1)) + cos(chi_q) * (p(2) - r(2));
    chi_c = chi_q - chi_inf*2/pi * atan(k_path*e_crosstrack);
elseif strcmp(path_struct.type,'orb')
    % Implement the orbit path follower
    % Algorithm 4
    % Center = [Cn; Ce; Cd]
    
    h_c = -center(3);
    d = sqrt((p(1)-center(1))^2 + (p(2)-center(2))^2);
    swirl = atan2(p(2)-center(2), p(1)-center(1));
    while swirl - chi < pi
        swirl = swirl+2*pi;
        break
    end
    while swirl - chi > pi
        swirl = swirl-2*pi;
        break
    end
    chi_c = swirl + orbit_direction*(pi/2 + atan(k_orbit*((d-radius)/radius)));
    e_crosstrack = nan;
    test = 't';
else
    e_crosstrack = nan;
    chi_c = calc_chi(state);
    h_c = -state(3);
end
